simulink model "Bipolar_PWM_Single_Phase_Inverter"  (R2025a)
settings: Solver=ode23tb  StartTime=0.0  StopTime=0.1  MaxStep=1e-4  RelTol=1e-3
libraries: spsIGBTDiodeLib x4, spsSawtoothGeneratorLib x2, spsRMSLib x1, spsSeriesRLCBranchLib x1, spsVoltageMeasurementLib x1, spsDCVoltageSourceLib x1, sps_lib x1
settings Model: Creator=Jawad  LastModifiedBy=Jawad

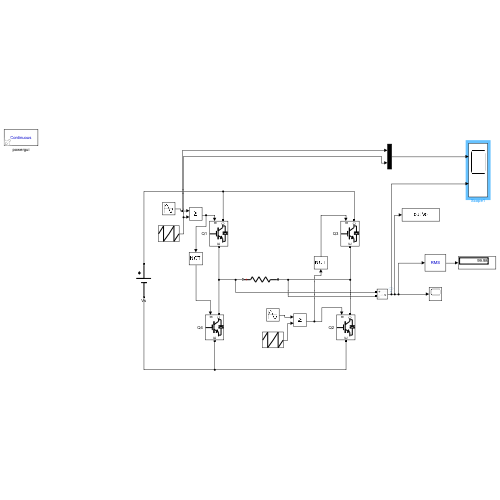
[thumbnail: Simulink's stored preview of the top-level diagram]
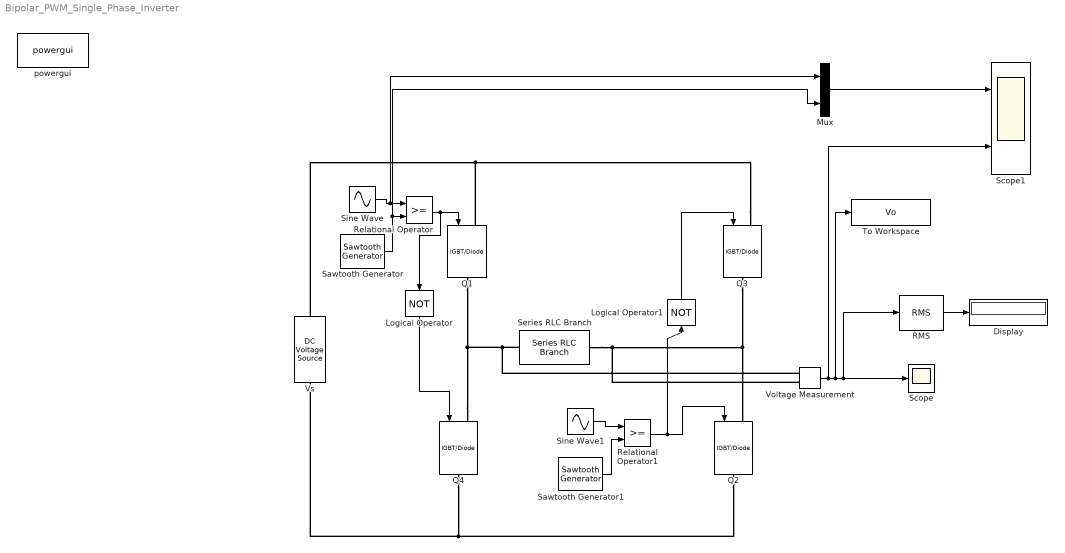
== system Bipolar_PWM_Single_Phase_Inverter ==
  Display : Display
  Logical Operator : Logic  Operator=NOT  AllPortsSameDT=off  OutDataTypeStr=boolean
  Logical Operator1 : Logic  Operator=NOT  AllPortsSameDT=off  OutDataTypeStr=boolean
  Mux : Mux  Inputs=2
  Q{1..4} (4 alike) : spsIGBTDiodeLib/IGBT//Diode  Ron=1e-3  Rs=1e5  Cs=inf  Measurements=off
  RMS : spsRMSLib/RMS  TrueRMS=on  Freq=60  RMSInit=120  Ts=0
  Relational Operator : RelationalOperator  OutDataTypeStr=boolean  RndMeth=Simplest  InputSameDT=off
  Relational Operator1 : RelationalOperator  OutDataTypeStr=boolean  RndMeth=Simplest  InputSameDT=off
  Sawtooth Generator : spsSawtoothGeneratorLib/Sawtooth Generator  Freq=1000  Phase=180  Ts=0
  Sawtooth Generator1 : spsSawtoothGeneratorLib/Sawtooth Generator  Freq=1000  Phase=180  Ts=0
  Scope : Scope
      settings: ActiveDisplayYMinimum=-124.97500249999995  ActiveDisplayYMaximum=124.97500249999995
  Scope1 : Scope  NumInputPorts=2
      settings: ActiveDisplayYMinimum=-1.1444567623000963  ActiveDisplayYMaximum=1.355543237699872
  Series RLC Branch : spsSeriesRLCBranchLib/Series RLC Branch  LConnTagsString=__new0  RConnTagsString=__new0  BranchType=R  Resistance=10  Inductance=1e-3  SetiL0=off  InitialCurrent=0  Capacitance=1e-6  Setx0=off  InitialVoltage=0  Measurements=None
  Sine Wave : Sin  Amplitude=0.8  Frequency=2*pi*50  SampleTime=0
  Sine Wave1 : Sin  Amplitude=0.8  Frequency=2*pi*50  SampleTime=0
  To Workspace : ToWorkspace  VariableName=Vo  SaveFormat=Structure With Time  SampleTime=-1
  Voltage Measurement : spsVoltageMeasurementLib/Voltage Measurement  PhasorSimulation=off  OutputType=Complex  PSBequivalent=0
  Vs : spsDCVoltageSourceLib/DC Voltage Source  Amplitude=100  Measurements=None
  powergui : sps_lib/powergui  Priority=1  SimulationMode=Continuous  SampleTime=50e-6  frequency=60  Iterations=50  frequencyindice=0  Pbase=100e6  ErrMax=1e-4  UnitsV=kV  UnitsW=MW  buscounter=0  FunctionMessages=off  echomessages=off  EnableUseOfTLC=off  CurrentSourceSwitches=off  DisableSnubberDevices=off  DisableRonSwitches=off  DisableVfSwitches=off  DisplayEquations=off  AutomaticDiscreteSolvers=off  SolverType=Tustin/Backward Euler (TBE)  Interpol=off  ExternalGateDelay=off  methode=off  Ts=100  x0status=blocks  SPID=on  SwTol=0  HookPort=off  NonlinearTolerance=1e-4  nMaxIteration=100  ContinueOnMaxIteration=off  RestoreLinks=warning  ResistiveCurrentMeasurement=off  Frange=[0:2:500]  Ylog=off  Xlog=on  ShowGrid=off  save=off  variable=ZData  structure=0  ZoomFFT=off  StartTime=0.0  cycles=1  DisplayStyle=1  fundamental=60  FreqAxis=off  MaxFrequency=1000  frequencyindicesteady=1  RmsSteady=1  display=off
  wires:
  RMS/1 -> Display/1
  Voltage Measurement/1 -> Scope1/2, To Workspace/1, RMS/1, Scope/1
  Sawtooth Generator/1 -> Mux/2, Relational Operator/2
  Relational Operator/1 -> Q1/1, Logical Operator/1
  Logical Operator/1 -> Q4/1
  Sine Wave1/1 -> Relational Operator1/1
  Sawtooth Generator1/1 -> Relational Operator1/2
  Relational Operator1/1 -> Q2/1, Logical Operator1/1
  Logical Operator1/1 -> Q3/1
  Sine Wave/1 -> Mux/1, Relational Operator/1
  Mux/1 -> Scope1/1
  connections:
  Vs/LConn1 -- Q2/RConn1 -- Q4/RConn1
  Series RLC Branch/RConn1 -- Q3/RConn1 -- Q2/LConn1 -- Voltage Measurement/LConn2
  Q3/LConn1 -- Vs/RConn1 -- Q1/LConn1
  Q4/LConn1 -- Q1/RConn1 -- Voltage Measurement/LConn1 -- Series RLC Branch/LConn1
